simulink model "Parametrica"  (R2020b)
settings: Solver=VariableStepAuto  StartTime=0.0  StopTime=Smi.general.simulation_time  FixedStep=0.001  MaxStep=0.001  RelTol=1e-3  AbsTol=1e-3  EnableMultiTasking=on
undefined symbols (not defined in the file): Smi, X, Y, Z
libraries: sm_lib x754, nesl_utility x195, simulink x10, cstblocks x8, dspsrcs4 x6
(part 1 of 26)
settings Model: Creator=nicop  LastModifiedBy=lemon
settings SolverCC: AutoScaleAbsTol=off
settings DataIOCC: LimitDataPoints=on  MaxDataPoints=10000
settings OptimizationCC: LifeSpan=inf
settings DebuggingCC: ReadBeforeWriteMsg=DisableAll  WriteAfterWriteMsg=DisableAll  WriteAfterReadMsg=DisableAll  MultiTaskDSMMsg=none  AllowSymbolicDim=off  SFUnexpectedBacktrackingDiag=warning  SFNoUnconditionalDefaultTransitionDiag=warning  SFExecutionAtInitializationDiag=none  ArithmeticOperatorsInVariantConditions=warning
settings SFSimCC: SFSimEcho=off  SimUseLocalCustomCode=off  CustomCodeUndefinedFunction=UseInterfaceOnly
settings RTWCC: RTWUseLocalCustomCode=off
settings CodeAppCC: StateflowObjectComments=on
settings GRTTargetCC: TargetLangStandard=C89/C90 (ANSI)
settings ConfigComp: CovMetricSettings=dw  CovSaveCumulativeToWorkspaceVar=on  CovSaveSingleToWorkspaceVar=on  CovExternalEMLEnable=off  CovSFcnEnable=off
settings SimscapeCC: SimscapeLogType=all  SimscapeLogSimulationStatistics=on  SimscapeLogDataHistory=10000

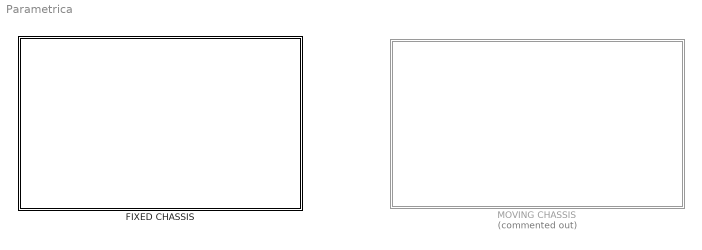
== system Parametrica ==
  FIXED CHASSIS : Subsystem
  MOVING CHASSIS : Subsystem  Commented=on

== system Parametrica/FIXED CHASSIS ==
  ACTUATOR FL : Subsystem
  ACTUATOR FR : Subsystem
  ACTUATOR RL : Subsystem  Commented=on
  ACTUATOR RR : Subsystem  Commented=on
  ARB FORCE FRONT : Subsystem
      settings: PortSchema="{\"entries\":[{\"content\":{\"sides\":[{\"content\":{\"connectorIds\":[\"In1\"]},\"type\":\"ConnectorPlacement.EquallySpacedRectSide\",\"uuid\":\"f25b79aa-b224-4593-8684-6f41613af52b\"},{\"content\":{\"connectorIds\":[\"In2\"],\"side\":\"RIGHT\"},\"type\":\"ConnectorPlacement.EquallySpacedRectSide\",\"uuid\":\"26f4e7e1-091e-45ed-9f78-3987c8995f75\"},{\"content\":{\"connectorIds\":[],\"side\":\"TOP\"},\"type\":\"ConnectorPlacement.EquallySpacedRectSide\",\"uuid\":\"90235f4e-ba57-4fcb-bbd6-69b42c3c6a9e\"},{\"content\":{\"connectorIds\":[\"RConn1\"],\"side\":\"BOTTOM\"},\"type\":\"ConnectorPlacement.EquallySpacedRectSide\",\"uuid\":\"3db937b0-450c-45c4-a882-0a0f348dea43\"},{\"content\":{\"connectorIds\":[],\"side\":\"HIDDEN\"},\"type\":\"ConnectorPlacement.EquallySpacedRectSide\",\"uuid\":\"b4049281-0224-45ee-bb5a-d89597eff6c9\"}]},\"type\":\"ConnectorPlacement.EquallySpacedConnector\",\"uuid\":\"c287e8ca-6e86-426d-a5dc-abeb0131b4c7\"}],\"packageUris\":[\"http://schema.mathworks.com/mf0/Connector/R2020b\"],\"version\":\"1.0\"}"
  ARB FORCE REAR : Subsystem  Commented=on
      settings: PortSchema="{\"entries\":[{\"content\":{\"sides\":[{\"content\":{\"connectorIds\":[\"In1\"]},\"type\":\"ConnectorPlacement.EquallySpacedRectSide\",\"uuid\":\"f25b79aa-b224-4593-8684-6f41613af52b\"},{\"content\":{\"connectorIds\":[\"In2\"],\"side\":\"RIGHT\"},\"type\":\"ConnectorPlacement.EquallySpacedRectSide\",\"uuid\":\"26f4e7e1-091e-45ed-9f78-3987c8995f75\"},{\"content\":{\"connectorIds\":[\"LConn1\"],\"side\":\"TOP\"},\"type\":\"ConnectorPlacement.EquallySpacedRectSide\",\"uuid\":\"90235f4e-ba57-4fcb-bbd6-69b42c3c6a9e\"},{\"content\":{\"connectorIds\":[],\"side\":\"BOTTOM\"},\"type\":\"ConnectorPlacement.EquallySpacedRectSide\",\"uuid\":\"3db937b0-450c-45c4-a882-0a0f348dea43\"},{\"content\":{\"connectorIds\":[],\"side\":\"HIDDEN\"},\"type\":\"ConnectorPlacement.EquallySpacedRectSide\",\"uuid\":\"b4049281-0224-45ee-bb5a-d89597eff6c9\"}]},\"type\":\"ConnectorPlacement.EquallySpacedConnector\",\"uuid\":\"c287e8ca-6e86-426d-a5dc-abeb0131b4c7\"}],\"packageUris\":[\"http://schema.mathworks.com/mf0/Connector/R2020b\"],\"version\":\"1.0\"}"
  BODY : Subsystem
      settings: PortSchema="{\"entries\":[{\"content\":{\"sides\":[{\"content\":{\"connectorIds\":[\"LConn1\",\"LConn2\",\"LConn3\",\"LConn4\",\"LConn5\",\"LConn6\",\"LConn7\",\"LConn8\",\"LConn9\",\"LConn10\",\"LConn11\",\"LConn12\",\"LConn13\",\"LConn14\",\"LConn15\",\"LConn16\",\"LConn17\",\"LConn18\"]},\"type\":\"ConnectorPlacement.EquallySpacedRectSide\",\"uuid\":\"4c2bbaf1-fbd8-4943-99e0-470de1938501\"},{\"content\":{\"connectorIds\":[\"RConn1\",\"RConn2\",\"RConn3\",\"RConn4\",\"RConn5\",\"RConn6\",\"RConn7\",\"RConn8\",\"RConn9\",\"RConn10\",\"RConn11\",\"RConn12\",\"RConn13\",\"RConn14\",\"RConn15\",\"RConn16\",\"RConn17\",\"RConn18\"],\"side\":\"RIGHT\"},\"type\":\"ConnectorPlacement.EquallySpacedRectSide\",\"uuid\":\"782ff682-1e99-4a86-9ae1-6b10d64c2634\"},{\"content\":{\"connectorIds\":[\"LConn19\"],\"side\":\"TOP\"},\"type\":\"ConnectorPlacement.EquallySpacedRectSide\",\"uuid\":\"0b3565bb-f882-4cc1-9f6f-7b6d6ef48850\"},{\"content\":{\"connectorIds\":[\"RConn19\"],\"side\":\"BOTTOM\"},\"type\":\"ConnectorPlacement.EquallySpacedRectSide\",\"uuid\":\"2660912b-114d-4160-a2f6-1b97c7cfb4a4\"},{\"content\":{\"connectorIds\":[],\"side\":\"HIDDEN\"},\"type\":\"ConnectorPlacement.EquallySpacedRectSide\",\"uuid\":\"29404510-5925-4bb6-a2d1-6f2b8f5e0381\"}]},\"type\":\"ConnectorPlacement.EquallySpacedConnector\",\"uuid\":\"2c55a6b1-9684-4292-96ca-1ed68c3a6f99\"}],\"packageUris\":[\"http://schema.mathworks.com/mf0/Connector/R2020b\"],\"version\":\"1.0\"}"
  FL SUSPENSION : Subsystem
  FR SUSPENSION : Subsystem
  RL SUSPENSION : Subsystem  Commented=on
      settings: PortSchema="{\"entries\":[{\"content\":{\"sides\":[{\"content\":{\"connectorIds\":[\"LConn1\",\"LConn2\"]},\"type\":\"ConnectorPlacement.EquallySpacedRectSide\",\"uuid\":\"871081ea-2c24-4d21-832e-5640a25161e2\"},{\"content\":{\"connectorIds\":[\"RConn1\",\"RConn2\",\"RConn3\",\"RConn4\",\"RConn5\",\"RConn6\",\"RConn7\",\"RConn8\",\"RConn9\",\"Out1\"],\"side\":\"RIGHT\"},\"type\":\"ConnectorPlacement.EquallySpacedRectSide\",\"uuid\":\"a664e2f3-4231-4f74-b53f-ae4988c7c2e0\"},{\"content\":{\"connectorIds\":[],\"side\":\"TOP\"},\"type\":\"ConnectorPlacement.EquallySpacedRectSide\",\"uuid\":\"bdace652-9708-4907-99cc-0edabcb09431\"},{\"content\":{\"connectorIds\":[],\"side\":\"HIDDEN\"},\"type\":\"ConnectorPlacement.EquallySpacedRectSide\",\"uuid\":\"50ce3595-7239-4383-a258-2477be36e9ad\"}]},\"type\":\"ConnectorPlacement.EquallySpacedConnector\",\"uuid\":\"d496f71a-4c83-49fc-a377-4524f909a5a7\"}],\"packageUris\":[\"http://schema.mathworks.com/mf0/Connector/R2020b\"],\"version\":\"1.0\"}"
  RR SUSPENSION : Subsystem  Commented=on
      settings: PortSchema="{\"entries\":[{\"content\":{\"sides\":[{\"content\":{\"connectorIds\":[\"LConn1\",\"LConn2\"]},\"type\":\"ConnectorPlacement.EquallySpacedRectSide\",\"uuid\":\"871081ea-2c24-4d21-832e-5640a25161e2\"},{\"content\":{\"connectorIds\":[\"RConn1\",\"RConn2\",\"RConn3\",\"RConn4\",\"RConn5\",\"RConn6\",\"RConn7\",\"RConn8\",\"RConn9\",\"Out1\"],\"side\":\"RIGHT\"},\"type\":\"ConnectorPlacement.EquallySpacedRectSide\",\"uuid\":\"a664e2f3-4231-4f74-b53f-ae4988c7c2e0\"},{\"content\":{\"connectorIds\":[],\"side\":\"TOP\"},\"type\":\"ConnectorPlacement.EquallySpacedRectSide\",\"uuid\":\"bdace652-9708-4907-99cc-0edabcb09431\"},{\"content\":{\"connectorIds\":[],\"side\":\"HIDDEN\"},\"type\":\"ConnectorPlacement.EquallySpacedRectSide\",\"uuid\":\"50ce3595-7239-4383-a258-2477be36e9ad\"}]},\"type\":\"ConnectorPlacement.EquallySpacedConnector\",\"uuid\":\"d496f71a-4c83-49fc-a377-4524f909a5a7\"}],\"packageUris\":[\"http://schema.mathworks.com/mf0/Connector/R2020b\"],\"version\":\"1.0\"}"
  WORLD : Subsystem
  wires:
  FR SUSPENSION/1(ARB ANGLE) -> ARB FORCE FRONT/2(ARB° RIGHT)
  RL SUSPENSION/1(ARB ANGLE) -> ARB FORCE REAR/1(ARB° LEFT)
  RR SUSPENSION/1(ARB ANGLE) -> ARB FORCE REAR/2(ARB° RIGHT)
  FL SUSPENSION/1(ARB ANGLE) -> ARB FORCE FRONT/1(ARB° LEFT)
  connections:
  BODY/RConn3 -- FR SUSPENSION/RConn5
  RR SUSPENSION/RConn8 -- BODY/RConn18
  BODY/LConn7 -- FL SUSPENSION/RConn9
  ARB FORCE FRONT/RConn1 -- FR SUSPENSION/RConn1 -- FL SUSPENSION/RConn1
  RR SUSPENSION/RConn5 -- BODY/RConn15
  FL SUSPENSION/RConn6 -- BODY/LConn4
  BODY/RConn2 -- FR SUSPENSION/RConn4
  BODY/LConn17 -- RL SUSPENSION/RConn7
  FL SUSPENSION/RConn5 -- BODY/LConn3
  ACTUATOR FR/LConn2 -- FR SUSPENSION/LConn1
  RL SUSPENSION/LConn1 -- ACTUATOR RL/LConn2
  RL SUSPENSION/RConn1 -- BODY/LConn11
  FL SUSPENSION/LConn2 -- ACTUATOR FL/LConn1
  FL SUSPENSION/RConn8 -- BODY/LConn6
  BODY/LConn9 -- ACTUATOR FL/RConn1
  ACTUATOR RL/LConn1 -- RL SUSPENSION/LConn2
  WORLD/RConn1 -- BODY/RConn19
  ACTUATOR RR/LConn1 -- RR SUSPENSION/LConn2
  FL SUSPENSION/RConn3 -- BODY/LConn1
  BODY/LConn19 -- FR SUSPENSION/RConn2 -- FL SUSPENSION/RConn2
  BODY/RConn4 -- FR SUSPENSION/RConn6
  RR SUSPENSION/RConn3 -- BODY/RConn13
  BODY/LConn5 -- FL SUSPENSION/RConn7
  BODY/RConn5 -- FR SUSPENSION/RConn7
  BODY/RConn1 -- FR SUSPENSION/RConn3
  RR SUSPENSION/RConn6 -- BODY/RConn16
  BODY/LConn12 -- RL SUSPENSION/RConn2
  BODY/RConn7 -- FR SUSPENSION/RConn9
  RR SUSPENSION/RConn4 -- BODY/RConn14
  RR SUSPENSION/RConn2 -- BODY/RConn12
  BODY/RConn6 -- FR SUSPENSION/RConn8
  BODY/LConn16 -- RL SUSPENSION/RConn6
  FL SUSPENSION/RConn4 -- BODY/LConn2
  RR SUSPENSION/RConn1 -- BODY/RConn11
  BODY/LConn14 -- RL SUSPENSION/RConn4
  RR SUSPENSION/RConn7 -- BODY/RConn17
  BODY/RConn8 -- FR SUSPENSION/RConn10
  BODY/LConn10 -- ACTUATOR RL/RConn1
  BODY/RConn9 -- ACTUATOR FR/RConn1
  ARB FORCE REAR/LConn1 -- RR SUSPENSION/RConn9 -- RL SUSPENSION/RConn9
  RL SUSPENSION/RConn3 -- BODY/LConn13
  BODY/RConn10 -- ACTUATOR RR/RConn1
  FL SUSPENSION/RConn10 -- BODY/LConn8
  RR SUSPENSION/LConn1 -- ACTUATOR RR/LConn2
  BODY/LConn18 -- RL SUSPENSION/RConn8
  ACTUATOR FL/LConn2 -- FL SUSPENSION/LConn1
  FR SUSPENSION/LConn2 -- ACTUATOR FR/LConn1
  RL SUSPENSION/RConn5 -- BODY/LConn15

== system Parametrica/MOVING CHASSIS ==
  ACTUATOR FL : Subsystem
  ACTUATOR FR : Subsystem
  ACTUATOR RL : Subsystem
  ACTUATOR RR : Subsystem
  ARB FORCE FRONT1 : Subsystem
      settings: PortSchema="{\"entries\":[{\"content\":{\"sides\":[{\"content\":{\"connectorIds\":[\"In1\"]},\"type\":\"ConnectorPlacement.EquallySpacedRectSide\",\"uuid\":\"f25b79aa-b224-4593-8684-6f41613af52b\"},{\"content\":{\"connectorIds\":[\"In2\"],\"side\":\"RIGHT\"},\"type\":\"ConnectorPlacement.EquallySpacedRectSide\",\"uuid\":\"26f4e7e1-091e-45ed-9f78-3987c8995f75\"},{\"content\":{\"connectorIds\":[],\"side\":\"TOP\"},\"type\":\"ConnectorPlacement.EquallySpacedRectSide\",\"uuid\":\"90235f4e-ba57-4fcb-bbd6-69b42c3c6a9e\"},{\"content\":{\"connectorIds\":[\"RConn1\"],\"side\":\"BOTTOM\"},\"type\":\"ConnectorPlacement.EquallySpacedRectSide\",\"uuid\":\"3db937b0-450c-45c4-a882-0a0f348dea43\"},{\"content\":{\"connectorIds\":[],\"side\":\"HIDDEN\"},\"type\":\"ConnectorPlacement.EquallySpacedRectSide\",\"uuid\":\"b4049281-0224-45ee-bb5a-d89597eff6c9\"}]},\"type\":\"ConnectorPlacement.EquallySpacedConnector\",\"uuid\":\"c287e8ca-6e86-426d-a5dc-abeb0131b4c7\"}],\"packageUris\":[\"http://schema.mathworks.com/mf0/Connector/R2020b\"],\"version\":\"1.0\"}"
  ARB FORCE REAR : Subsystem
      settings: PortSchema="{\"entries\":[{\"content\":{\"sides\":[{\"content\":{\"connectorIds\":[\"In1\"]},\"type\":\"ConnectorPlacement.EquallySpacedRectSide\",\"uuid\":\"f25b79aa-b224-4593-8684-6f41613af52b\"},{\"content\":{\"connectorIds\":[\"In2\"],\"side\":\"RIGHT\"},\"type\":\"ConnectorPlacement.EquallySpacedRectSide\",\"uuid\":\"26f4e7e1-091e-45ed-9f78-3987c8995f75\"},{\"content\":{\"connectorIds\":[\"LConn1\"],\"side\":\"TOP\"},\"type\":\"ConnectorPlacement.EquallySpacedRectSide\",\"uuid\":\"90235f4e-ba57-4fcb-bbd6-69b42c3c6a9e\"},{\"content\":{\"connectorIds\":[],\"side\":\"BOTTOM\"},\"type\":\"ConnectorPlacement.EquallySpacedRectSide\",\"uuid\":\"3db937b0-450c-45c4-a882-0a0f348dea43\"},{\"content\":{\"connectorIds\":[],\"side\":\"HIDDEN\"},\"type\":\"ConnectorPlacement.EquallySpacedRectSide\",\"uuid\":\"b4049281-0224-45ee-bb5a-d89597eff6c9\"}]},\"type\":\"ConnectorPlacement.EquallySpacedConnector\",\"uuid\":\"c287e8ca-6e86-426d-a5dc-abeb0131b4c7\"}],\"packageUris\":[\"http://schema.mathworks.com/mf0/Connector/R2020b\"],\"version\":\"1.0\"}"
  BODY : Subsystem
      settings: PortSchema="{\"entries\":[{\"content\":{\"sides\":[{\"content\":{\"connectorIds\":[\"LConn1\",\"LConn2\",\"LConn3\",\"LConn4\",\"LConn5\",\"LConn6\",\"LConn7\",\"LConn8\",\"LConn9\",\"LConn10\",\"LConn11\",\"LConn12\",\"LConn13\",\"LConn14\",\"LConn15\",\"LConn16\"]},\"type\":\"ConnectorPlacement.EquallySpacedRectSide\",\"uuid\":\"4c2bbaf1-fbd8-4943-99e0-470de1938501\"},{\"content\":{\"connectorIds\":[\"RConn1\",\"RConn2\",\"RConn3\",\"RConn4\",\"RConn5\",\"RConn6\",\"RConn7\",\"RConn8\",\"RConn9\",\"RConn10\",\"RConn11\",\"RConn12\",\"RConn13\",\"RConn14\",\"RConn15\",\"RConn16\"],\"side\":\"RIGHT\"},\"type\":\"ConnectorPlacement.EquallySpacedRectSide\",\"uuid\":\"782ff682-1e99-4a86-9ae1-6b10d64c2634\"},{\"content\":{\"connectorIds\":[\"LConn17\"],\"side\":\"TOP\"},\"type\":\"ConnectorPlacement.EquallySpacedRectSide\",\"uuid\":\"0b3565bb-f882-4cc1-9f6f-7b6d6ef48850\"},{\"content\":{\"connectorIds\":[\"RConn17\"],\"side\":\"BOTTOM\"},\"type\":\"ConnectorPlacement.EquallySpacedRectSide\",\"uuid\":\"2660912b-114d-4160-a2f6-1b97c7cfb4a4\"},{\"content\":{\"connectorIds\":[],\"side\":\"HIDDEN\"},\"type\":\"ConnectorPlacement.EquallySpacedRectSide\",\"uuid\":\"29404510-5925-4bb6-a2d1-6f2b8f5e0381\"}]},\"type\":\"ConnectorPlacement.EquallySpacedConnector\",\"uuid\":\"2c55a6b1-9684-4292-96ca-1ed68c3a6f99\"}],\"packageUris\":[\"http://schema.mathworks.com/mf0/Connector/R2020b\"],\"version\":\"1.0\"}"
  FIXED ACTUATORS : Subsystem
      settings: PortSchema="{\"entries\":[{\"content\":{\"sides\":[{\"content\":{\"connectorIds\":[\"LConn1\",\"LConn2\"]},\"type\":\"ConnectorPlacement.EquallySpacedRectSide\",\"uuid\":\"4c2bbaf1-fbd8-4943-99e0-470de1938501\"},{\"content\":{\"connectorIds\":[\"RConn1\",\"RConn2\"],\"side\":\"RIGHT\"},\"type\":\"ConnectorPlacement.EquallySpacedRectSide\",\"uuid\":\"782ff682-1e99-4a86-9ae1-6b10d64c2634\"},{\"content\":{\"connectorIds\":[],\"side\":\"TOP\"},\"type\":\"ConnectorPlacement.EquallySpacedRectSide\",\"uuid\":\"0b3565bb-f882-4cc1-9f6f-7b6d6ef48850\"},{\"content\":{\"connectorIds\":[\"RConn3\"],\"side\":\"BOTTOM\"},\"type\":\"ConnectorPlacement.EquallySpacedRectSide\",\"uuid\":\"2660912b-114d-4160-a2f6-1b97c7cfb4a4\"},{\"content\":{\"connectorIds\":[],\"side\":\"HIDDEN\"},\"type\":\"ConnectorPlacement.EquallySpacedRectSide\",\"uuid\":\"29404510-5925-4bb6-a2d1-6f2b8f5e0381\"}]},\"type\":\"ConnectorPlacement.EquallySpacedConnector\",\"uuid\":\"2c55a6b1-9684-4292-96ca-1ed68c3a6f99\"}],\"packageUris\":[\"http://schema.mathworks.com/mf0/Connector/R2020b\"],\"version\":\"1.0\"}"
  FL SUSPENSION : Subsystem
  FR SUSPENSION : Subsystem
  RL SUSPENSION : Subsystem
      settings: PortSchema="{\"entries\":[{\"content\":{\"sides\":[{\"content\":{\"connectorIds\":[\"LConn1\",\"LConn2\"]},\"type\":\"ConnectorPlacement.EquallySpacedRectSide\",\"uuid\":\"871081ea-2c24-4d21-832e-5640a25161e2\"},{\"content\":{\"connectorIds\":[\"RConn1\",\"RConn2\",\"RConn3\",\"RConn4\",\"RConn5\",\"RConn6\",\"RConn7\",\"RConn8\",\"RConn9\",\"Out1\"],\"side\":\"RIGHT\"},\"type\":\"ConnectorPlacement.EquallySpacedRectSide\",\"uuid\":\"a664e2f3-4231-4f74-b53f-ae4988c7c2e0\"},{\"content\":{\"connectorIds\":[],\"side\":\"TOP\"},\"type\":\"ConnectorPlacement.EquallySpacedRectSide\",\"uuid\":\"bdace652-9708-4907-99cc-0edabcb09431\"},{\"content\":{\"connectorIds\":[],\"side\":\"HIDDEN\"},\"type\":\"ConnectorPlacement.EquallySpacedRectSide\",\"uuid\":\"50ce3595-7239-4383-a258-2477be36e9ad\"}]},\"type\":\"ConnectorPlacement.EquallySpacedConnector\",\"uuid\":\"d496f71a-4c83-49fc-a377-4524f909a5a7\"}],\"packageUris\":[\"http://schema.mathworks.com/mf0/Connector/R2020b\"],\"version\":\"1.0\"}"
  RR SUSPENSION : Subsystem
      settings: PortSchema="{\"entries\":[{\"content\":{\"sides\":[{\"content\":{\"connectorIds\":[\"LConn1\",\"LConn2\"]},\"type\":\"ConnectorPlacement.EquallySpacedRectSide\",\"uuid\":\"871081ea-2c24-4d21-832e-5640a25161e2\"},{\"content\":{\"connectorIds\":[\"RConn1\",\"RConn2\",\"RConn3\",\"RConn4\",\"RConn5\",\"RConn6\",\"RConn7\",\"RConn8\",\"RConn9\",\"Out1\"],\"side\":\"RIGHT\"},\"type\":\"ConnectorPlacement.EquallySpacedRectSide\",\"uuid\":\"a664e2f3-4231-4f74-b53f-ae4988c7c2e0\"},{\"content\":{\"connectorIds\":[],\"side\":\"TOP\"},\"type\":\"ConnectorPlacement.EquallySpacedRectSide\",\"uuid\":\"bdace652-9708-4907-99cc-0edabcb09431\"},{\"content\":{\"connectorIds\":[],\"side\":\"HIDDEN\"},\"type\":\"ConnectorPlacement.EquallySpacedRectSide\",\"uuid\":\"50ce3595-7239-4383-a258-2477be36e9ad\"}]},\"type\":\"ConnectorPlacement.EquallySpacedConnector\",\"uuid\":\"d496f71a-4c83-49fc-a377-4524f909a5a7\"}],\"packageUris\":[\"http://schema.mathworks.com/mf0/Connector/R2020b\"],\"version\":\"1.0\"}"
  WORLD : Subsystem
  wires:
  RR SUSPENSION/1(ARB ANGLE) -> ARB FORCE REAR/2(ARB° RIGHT)
  RL SUSPENSION/1(ARB ANGLE) -> ARB FORCE REAR/1(ARB° LEFT)
  FR SUSPENSION/1(ARB ANGLE) -> ARB FORCE FRONT1/2(ARB° RIGHT)
  FL SUSPENSION/1(ARB ANGLE) -> ARB FORCE FRONT1/1(ARB° LEFT)
  connections:
  FIXED ACTUATORS/RConn3 -- WORLD/RConn1 -- BODY/RConn17
  ACTUATOR RR/RConn1 -- FIXED ACTUATORS/RConn1
  ACTUATOR FL/RConn1 -- FIXED ACTUATORS/LConn2
  BODY/RConn1 -- FR SUSPENSION/RConn3
  FIXED ACTUATORS/LConn1 -- ACTUATOR RL/RConn1
  ACTUATOR RR/LConn2 -- RR SUSPENSION/LConn1
  BODY/RConn5 -- FR SUSPENSION/RConn7
  RR SUSPENSION/RConn8 -- BODY/RConn16
  BODY/LConn15 -- RL SUSPENSION/RConn7
  BODY/RConn7 -- FR SUSPENSION/RConn9
  BODY/RConn8 -- FR SUSPENSION/RConn10
  FL SUSPENSION/RConn10 -- BODY/LConn8
  RR SUSPENSION/RConn1 -- BODY/RConn9
  BODY/LConn16 -- RL SUSPENSION/RConn8
  RR SUSPENSION/RConn7 -- BODY/RConn15
  ACTUATOR FR/RConn1 -- FIXED ACTUATORS/RConn2
  BODY/RConn2 -- FR SUSPENSION/RConn4
  FL SUSPENSION/RConn6 -- BODY/LConn4
  BODY/LConn14 -- RL SUSPENSION/RConn6
  ACTUATOR RR/LConn1 -- RR SUSPENSION/LConn2
  RR SUSPENSION/RConn3 -- BODY/RConn11
  RR SUSPENSION/RConn6 -- BODY/RConn14
  RL SUSPENSION/LConn2 -- ACTUATOR RL/LConn1
  RL SUSPENSION/RConn3 -- BODY/LConn11
  ACTUATOR RL/LConn2 -- RL SUSPENSION/LConn1
  ACTUATOR FL/LConn2 -- FL SUSPENSION/LConn1
  BODY/RConn4 -- FR SUSPENSION/RConn6
  BODY/LConn5 -- FL SUSPENSION/RConn7
  BODY/LConn10 -- RL SUSPENSION/RConn2
  RL SUSPENSION/RConn1 -- BODY/LConn9
  ACTUATOR FR/LConn2 -- FR SUSPENSION/LConn1
  RR SUSPENSION/RConn5 -- BODY/RConn13
  RL SUSPENSION/RConn5 -- BODY/LConn13
  FL SUSPENSION/RConn1 -- ARB FORCE FRONT1/RConn1 -- FR SUSPENSION/RConn1
  FL SUSPENSION/RConn4 -- BODY/LConn2
  FL SUSPENSION/RConn2 -- BODY/LConn17 -- FR SUSPENSION/RConn2
  RR SUSPENSION/RConn2 -- BODY/RConn10
  RL SUSPENSION/RConn9 -- ARB FORCE REAR/LConn1 -- RR SUSPENSION/RConn9
  BODY/LConn12 -- RL SUSPENSION/RConn4
  BODY/LConn7 -- FL SUSPENSION/RConn9
  FL SUSPENSION/RConn5 -- BODY/LConn3
  ACTUATOR FR/LConn1 -- FR SUSPENSION/LConn2
  FL SUSPENSION/RConn8 -- BODY/LConn6
  BODY/RConn6 -- FR SUSPENSION/RConn8
  FL SUSPENSION/LConn2 -- ACTUATOR FL/LConn1
  RR SUSPENSION/RConn4 -- BODY/RConn12
  BODY/RConn3 -- FR SUSPENSION/RConn5
  FL SUSPENSION/RConn3 -- BODY/LConn1

== system Parametrica/FIXED CHASSIS/ACTUATOR FL ==
  ACTUATOR : Subsystem
  ACTUATOR IN/OUT : Subsystem
  Full geometry : PMIOPort  Side=Left
  WORLD : PMIOPort  Port=2  Side=Right
  CP : PMIOPort  Port=3  Side=Left
  connections:
  ACTUATOR/LConn2 -- CP/RConn1
  ACTUATOR/LConn1 -- Full geometry/RConn1
  ACTUATOR IN/OUT/LConn1 -- ACTUATOR/RConn1
  ACTUATOR IN/OUT/RConn1 -- WORLD/RConn1

== system Parametrica/FIXED CHASSIS/ACTUATOR FR ==
  ACTUATOR : Subsystem
  ACTUATOR IN/OUT : Subsystem
  OUTER ACTUATOR : Subsystem
      settings: PortSchema="{\"entries\":[{\"content\":{\"sides\":[{\"content\":{\"connectorIds\":[]},\"type\":\"ConnectorPlacement.EquallySpacedRectSide\",\"uuid\":\"d7e62bfe-6450-4a39-85d3-bed3049c321c\"},{\"content\":{\"connectorIds\":[],\"side\":\"RIGHT\"},\"type\":\"ConnectorPlacement.EquallySpacedRectSide\",\"uuid\":\"3cbc563a-0112-4986-bd57-0cf817b4d4bf\"},{\"content\":{\"connectorIds\":[\"LConn1\"],\"side\":\"TOP\"},\"type\":\"ConnectorPlacement.EquallySpacedRectSide\",\"uuid\":\"eb91a932-1d66-4430-a168-6ec694e02ce0\"},{\"content\":{\"connectorIds\":[\"RConn1\"],\"side\":\"BOTTOM\"},\"type\":\"ConnectorPlacement.EquallySpacedRectSide\",\"uuid\":\"a5a9eb1a-4070-480d-a72b-be2caa4d4ddd\"},{\"content\":{\"connectorIds\":[],\"side\":\"HIDDEN\"},\"type\":\"ConnectorPlacement.EquallySpacedRectSide\",\"uuid\":\"1c33bc41-55ff-4930-aaf8-325eabd2d214\"}]},\"type\":\"ConnectorPlacement.EquallySpacedConnector\",\"uuid\":\"9fea4cfe-800a-4673-925c-b7963aa13243\"}],\"packageUris\":[\"http://schema.mathworks.com/mf0/Connector/R2020b\"],\"version\":\"1.0\"}"
  Full geometry : PMIOPort  Side=Left
  WORLD : PMIOPort  Port=2  Side=Right
  CP : PMIOPort  Port=3  Side=Left
  connections:
  WORLD/RConn1 -- OUTER ACTUATOR/RConn1
  ACTUATOR IN/OUT/LConn1 -- ACTUATOR/RConn1
  ACTUATOR/LConn1 -- Full geometry/RConn1
  ACTUATOR/LConn2 -- CP/RConn1
  OUTER ACTUATOR/LConn1 -- ACTUATOR IN/OUT/RConn1

== system Parametrica/FIXED CHASSIS/ACTUATOR RL ==
  ACTUATOR : Subsystem
  ACTUATOR IN/OUT : Subsystem
  OUTER ACTUATOR : Subsystem
      settings: PortSchema="{\"entries\":[{\"content\":{\"sides\":[{\"content\":{\"connectorIds\":[]},\"type\":\"ConnectorPlacement.EquallySpacedRectSide\",\"uuid\":\"d7e62bfe-6450-4a39-85d3-bed3049c321c\"},{\"content\":{\"connectorIds\":[],\"side\":\"RIGHT\"},\"type\":\"ConnectorPlacement.EquallySpacedRectSide\",\"uuid\":\"3cbc563a-0112-4986-bd57-0cf817b4d4bf\"},{\"content\":{\"connectorIds\":[\"LConn1\"],\"side\":\"TOP\"},\"type\":\"ConnectorPlacement.EquallySpacedRectSide\",\"uuid\":\"eb91a932-1d66-4430-a168-6ec694e02ce0\"},{\"content\":{\"connectorIds\":[\"RConn1\"],\"side\":\"BOTTOM\"},\"type\":\"ConnectorPlacement.EquallySpacedRectSide\",\"uuid\":\"a5a9eb1a-4070-480d-a72b-be2caa4d4ddd\"},{\"content\":{\"connectorIds\":[],\"side\":\"HIDDEN\"},\"type\":\"ConnectorPlacement.EquallySpacedRectSide\",\"uuid\":\"1c33bc41-55ff-4930-aaf8-325eabd2d214\"}]},\"type\":\"ConnectorPlacement.EquallySpacedConnector\",\"uuid\":\"9fea4cfe-800a-4673-925c-b7963aa13243\"}],\"packageUris\":[\"http://schema.mathworks.com/mf0/Connector/R2020b\"],\"version\":\"1.0\"}"
  CP : PMIOPort  Side=Left
  Full geometry : PMIOPort  Port=2  Side=Left
  WORLD : PMIOPort  Port=3  Side=Right
  connections:
  WORLD/RConn1 -- OUTER ACTUATOR/RConn1
  ACTUATOR IN/OUT/LConn1 -- ACTUATOR/RConn1
  ACTUATOR/LConn1 -- Full geometry/RConn1
  ACTUATOR/LConn2 -- CP/RConn1
  OUTER ACTUATOR/LConn1 -- ACTUATOR IN/OUT/RConn1

== system Parametrica/FIXED CHASSIS/ACTUATOR RR ==
  ACTUATOR : Subsystem
  ACTUATOR IN/OUT : Subsystem
  OUTER ACTUATOR : Subsystem
      settings: PortSchema="{\"entries\":[{\"content\":{\"sides\":[{\"content\":{\"connectorIds\":[]},\"type\":\"ConnectorPlacement.EquallySpacedRectSide\",\"uuid\":\"d7e62bfe-6450-4a39-85d3-bed3049c321c\"},{\"content\":{\"connectorIds\":[],\"side\":\"RIGHT\"},\"type\":\"ConnectorPlacement.EquallySpacedRectSide\",\"uuid\":\"3cbc563a-0112-4986-bd57-0cf817b4d4bf\"},{\"content\":{\"connectorIds\":[\"LConn1\"],\"side\":\"TOP\"},\"type\":\"ConnectorPlacement.EquallySpacedRectSide\",\"uuid\":\"eb91a932-1d66-4430-a168-6ec694e02ce0\"},{\"content\":{\"connectorIds\":[\"RConn1\"],\"side\":\"BOTTOM\"},\"type\":\"ConnectorPlacement.EquallySpacedRectSide\",\"uuid\":\"a5a9eb1a-4070-480d-a72b-be2caa4d4ddd\"},{\"content\":{\"connectorIds\":[],\"side\":\"HIDDEN\"},\"type\":\"ConnectorPlacement.EquallySpacedRectSide\",\"uuid\":\"1c33bc41-55ff-4930-aaf8-325eabd2d214\"}]},\"type\":\"ConnectorPlacement.EquallySpacedConnector\",\"uuid\":\"9fea4cfe-800a-4673-925c-b7963aa13243\"}],\"packageUris\":[\"http://schema.mathworks.com/mf0/Connector/R2020b\"],\"version\":\"1.0\"}"
  CP : PMIOPort  Side=Left
  Full geometry : PMIOPort  Port=2  Side=Left
  WORLD : PMIOPort  Port=3  Side=Right
  connections:
  OUTER ACTUATOR/LConn1 -- ACTUATOR IN/OUT/RConn1
  ACTUATOR/LConn2 -- CP/RConn1
  ACTUATOR/LConn1 -- Full geometry/RConn1
  ACTUATOR IN/OUT/LConn1 -- ACTUATOR/RConn1
  WORLD/RConn1 -- OUTER ACTUATOR/RConn1

== system Parametrica/FIXED CHASSIS/ARB FORCE FRONT ==
  ARB° LEFT : Inport
  ARB° RIGHT : Inport  Port=2
  Constant : Constant  Value=Smi.Car.FRONT.elastic.ARB_stiffness
  Product : Product
  Simulink-PS Converter : nesl_utility/Simulink-PS Converter  PhysicalDomain=network_engine_domain  SubClassName=ps_input  LeftPortType=input  RightPortType=output  PseudoPeriodic=off  Frequencies=[]  NoiseDistribution=none  NoiseParameters=[]  Unit=1  AffineConversion=off  FilteringAndDerivatives=provide  SimscapeFilterOrder=1  InputFilterTimeConstant=0.001  UdotUserProvided=0
  Sum : Sum  Inputs=+-
  ARB FORCE : PMIOPort  Side=Right
  wires:
  Sum/1 -> Product/1
  ARB° RIGHT/1 -> Sum/2
  ARB° LEFT/1 -> Sum/1
  Constant/1 -> Product/2
  Product/1 -> Simulink-PS Converter/1
  connections:
  ARB FORCE/RConn1 -- Simulink-PS Converter/RConn1

== system Parametrica/FIXED CHASSIS/ARB FORCE REAR ==
  ARB° LEFT : Inport
  ARB° RIGHT : Inport  Port=2
  Constant : Constant  Value=Smi.Car.REAR.elastic.ARB_stiffness
  Product : Product
  Simulink-PS Converter : nesl_utility/Simulink-PS Converter  PhysicalDomain=network_engine_domain  SubClassName=ps_input  LeftPortType=input  RightPortType=output  PseudoPeriodic=off  Frequencies=[]  NoiseDistribution=none  NoiseParameters=[]  Unit=1  AffineConversion=off  FilteringAndDerivatives=provide  SimscapeFilterOrder=1  InputFilterTimeConstant=0.001  UdotUserProvided=0
  Sum : Sum  Inputs=+-
  ARB FORCE : PMIOPort  Side=Left
  wires:
  Product/1 -> Simulink-PS Converter/1
  Constant/1 -> Product/2
  ARB° LEFT/1 -> Sum/1
  ARB° RIGHT/1 -> Sum/2
  Sum/1 -> Product/1
  connections:
  ARB FORCE/RConn1 -- Simulink-PS Converter/RConn1

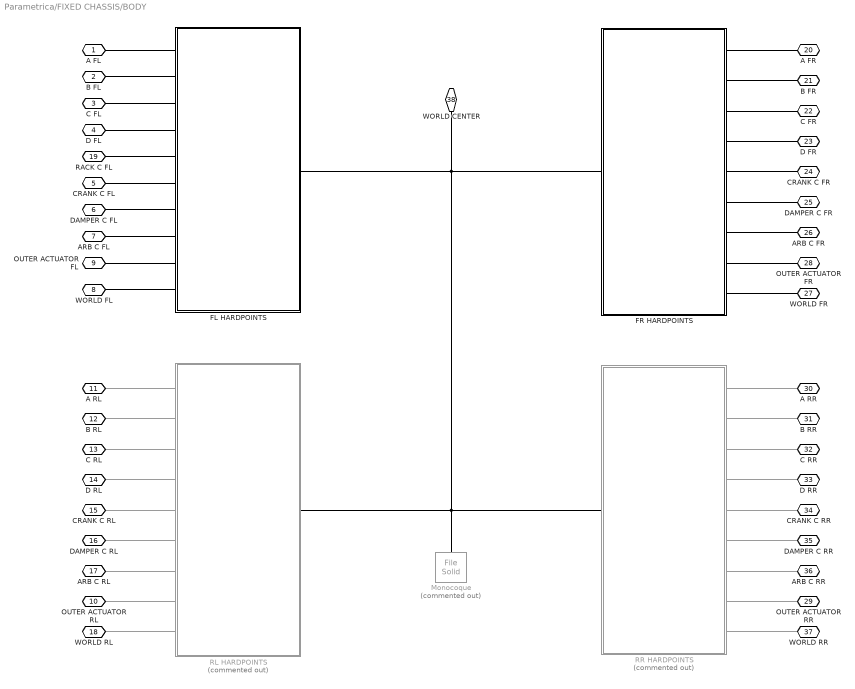
== system Parametrica/FIXED CHASSIS/BODY ==
  FL HARDPOINTS : Subsystem
  FR HARDPOINTS : Subsystem
  Monocoque : sm_lib/Body Elements/File Solid  Commented=on  ExtGeomFileName=Parameters\Monocoque.stp  UnitType=FromFile  ExtGeomFileUnits=m  StepReaderType=HEX  ExportConvexHullGeometry=off  InertiaType=PointMass  Mass=1  MassUnits=kg  CenterOfMass=[0 0 0]  CenterOfMassUnits=m  MomentsOfInertia=[1 1 1]  MomentsOfInertiaUnits=kg*m^2  ProductsOfInertia=[0 0 0]  ProductsOfInertiaUnits=kg*m^2  BasedOnType=DensityFromFile  Density=1000  DensityUnits=kg/m^3  DoExposeReferenceFrame=on  SerializedFrames=<Frames/>  GraphicType=FromGeometry  MarkerShape=Sphere  MarkerSize=10  GraphicVisPropType=SimpleVisualProperties  GraphicDiffuseColor=[1.0 1.0 1.0]  GraphicSpecularColor=[0.5 0.5 0.5 1.0]  GraphicAmbientColor=[0.15 0.15 0.15 1.0]  GraphicEmissiveColor=[0.0 0.0 0.0 1.0]  GraphicShininess=75  GraphicOpacity=0.4
  RL HARDPOINTS : Subsystem  Commented=on
  RR HARDPOINTS : Subsystem  Commented=on
  A FL : PMIOPort  Side=Left
  B FL : PMIOPort  Port=2  Side=Left
  C FL : PMIOPort  Port=3  Side=Left
  D FL : PMIOPort  Port=4  Side=Left
  CRANK C FL : PMIOPort  Port=5  Side=Left
  DAMPER C FL : PMIOPort  Port=6  Side=Left
  ARB C FL : PMIOPort  Port=7  Side=Left
  WORLD FL : PMIOPort  Port=8  Side=Left
  OUTER ACTUATOR FL : PMIOPort  Port=9  Side=Left
  OUTER ACTUATOR RL : PMIOPort  Port=10  Side=Left
  A RL : PMIOPort  Port=11  Side=Left
  B RL : PMIOPort  Port=12  Side=Left
  C RL : PMIOPort  Port=13  Side=Left
  D RL : PMIOPort  Port=14  Side=Left
  CRANK C RL : PMIOPort  Port=15  Side=Left
  DAMPER C RL : PMIOPort  Port=16  Side=Left
  ARB C RL : PMIOPort  Port=17  Side=Left
  WORLD RL : PMIOPort  Port=18  Side=Left
  RACK C FL : PMIOPort  Port=19  Side=Left
  A FR : PMIOPort  Port=20  Side=Right
  B FR : PMIOPort  Port=21  Side=Right
  C FR : PMIOPort  Port=22  Side=Right
  D FR : PMIOPort  Port=23  Side=Right
  CRANK C FR : PMIOPort  Port=24  Side=Right
  DAMPER C FR : PMIOPort  Port=25  Side=Right
  ARB C FR : PMIOPort  Port=26  Side=Right
  WORLD FR : PMIOPort  Port=27  Side=Right
  OUTER ACTUATOR FR : PMIOPort  Port=28  Side=Right
  OUTER ACTUATOR RR : PMIOPort  Port=29  Side=Right
  A RR : PMIOPort  Port=30  Side=Right
  B RR : PMIOPort  Port=31  Side=Right
  C RR : PMIOPort  Port=32  Side=Right
  D RR : PMIOPort  Port=33  Side=Right
  CRANK C RR : PMIOPort  Port=34  Side=Right
  DAMPER C RR : PMIOPort  Port=35  Side=Right
  ARB C RR : PMIOPort  Port=36  Side=Right
  WORLD RR : PMIOPort  Port=37  Side=Right
  WORLD CENTER : PMIOPort  Port=38  Side=Right
  connections:
  FL HARDPOINTS/RConn1 -- Monocoque/RConn1 -- RR HARDPOINTS/RConn1 -- RL HARDPOINTS/RConn1 -- FR HARDPOINTS/RConn1 -- WORLD CENTER/RConn1
  FL HARDPOINTS/LConn10 -- WORLD FL/RConn1
  OUTER ACTUATOR FL/RConn1 -- FL HARDPOINTS/LConn9
  FL HARDPOINTS/LConn8 -- ARB C FL/RConn1
  FL HARDPOINTS/LConn7 -- DAMPER C FL/RConn1
  FL HARDPOINTS/LConn6 -- CRANK C FL/RConn1
  RACK C FL/RConn1 -- FL HARDPOINTS/LConn5
  FL HARDPOINTS/LConn4 -- D FL/RConn1
  C FL/RConn1 -- FL HARDPOINTS/LConn3
  FL HARDPOINTS/LConn2 -- B FL/RConn1
  FL HARDPOINTS/LConn1 -- A FL/RConn1
  FR HARDPOINTS/LConn9 -- WORLD FR/RConn1
  FR HARDPOINTS/LConn8 -- OUTER ACTUATOR FR/RConn1
  FR HARDPOINTS/LConn7 -- ARB C FR/RConn1
  FR HARDPOINTS/LConn6 -- DAMPER C FR/RConn1
  FR HARDPOINTS/LConn5 -- CRANK C FR/RConn1
  FR HARDPOINTS/LConn3 -- C FR/RConn1
  FR HARDPOINTS/LConn4 -- D FR/RConn1
  B FR/RConn1 -- FR HARDPOINTS/LConn2
  FR HARDPOINTS/LConn1 -- A FR/RConn1
  RL HARDPOINTS/LConn2 -- B RL/RConn1
  RL HARDPOINTS/LConn1 -- A RL/RConn1
  RL HARDPOINTS/LConn3 -- C RL/RConn1
  RL HARDPOINTS/LConn4 -- D RL/RConn1
  RL HARDPOINTS/LConn5 -- CRANK C RL/RConn1
  RL HARDPOINTS/LConn6 -- DAMPER C RL/RConn1
  RL HARDPOINTS/LConn7 -- ARB C RL/RConn1
  RL HARDPOINTS/LConn8 -- OUTER ACTUATOR RL/RConn1
  RL HARDPOINTS/LConn9 -- WORLD RL/RConn1
  RR HARDPOINTS/LConn1 -- A RR/RConn1
  RR HARDPOINTS/LConn2 -- B RR/RConn1
  RR HARDPOINTS/LConn3 -- C RR/RConn1
  RR HARDPOINTS/LConn4 -- D RR/RConn1
  RR HARDPOINTS/LConn5 -- CRANK C RR/RConn1
  RR HARDPOINTS/LConn6 -- DAMPER C RR/RConn1
  RR HARDPOINTS/LConn7 -- ARB C RR/RConn1
  RR HARDPOINTS/LConn8 -- OUTER ACTUATOR RR/RConn1
  RR HARDPOINTS/LConn9 -- WORLD RR/RConn1
